simulink model "chap16_7sim"  (Simulink 8.3)
settings: Solver=ode45  StartTime=0.0  StopTime=10  FixedStep=0.001  RelTol=1e-3
settings Model: Creator=hp  LastModifiedBy=Administrator
settings DataIOCC: SignalLoggingName=sigsOut
settings OptimizationCC: ExpressionDepthLimit=2147483647  InitFltsAndDblsToZero=on
settings DebuggingCC: SaveWithParameterizedLinksMsg=none  SignalResolutionControl=TryResolveAllWithWarning  SolverPrmCheckMsg=none  MultiTaskDSMMsg=warning  MultiTaskCondExecSysMsg=none  FcnCallInpInsideContextMsg=UseLocalSettings
settings HardwareCC: TargetUnknown=on
settings RTWCC: IncludeERTFirstTime=on
settings GRTTargetCC: TargetFcnLib=ansi_tfl_tmw.mat

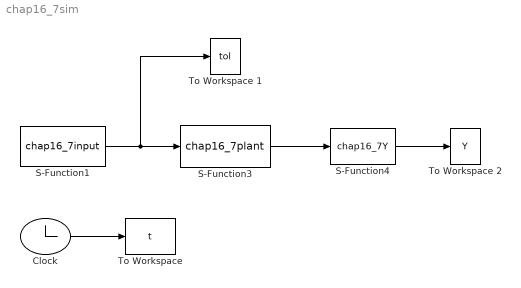
== system chap16_7sim ==
  Clock : Clock
  S-Function1 : S-Function  FunctionName=chap16_7input  EnableBusSupport=off
  S-Function3 : S-Function  FunctionName=chap16_7plant  EnableBusSupport=off
  S-Function4 : S-Function  FunctionName=chap16_7Y  EnableBusSupport=off
  To Workspace : ToWorkspace  VariableName=t  SampleTime=-1
  To Workspace 1 : ToWorkspace  VariableName=tol  SampleTime=-1
  To Workspace 2 : ToWorkspace  VariableName=Y  SampleTime=-1
  wires:
  Clock/1 -> To Workspace/1
  S-Function1/1 -> S-Function3/1, To Workspace 1/1
  S-Function3/1 -> S-Function4/1
  S-Function4/1 -> To Workspace 2/1
